simulink model "Opgave2_1"  (R2017a)
settings: Solver=VariableStepAuto  StartTime=0.0  StopTime=10.0  RelTol=1e-3
values from neighbouring files (symbols this model uses):
  b = 50    [Opgave2_1_script.m]
  F1 = 500    [Opgave2_1_script.m]
  m = 1000    [Opgave2_1_script.m]
settings Model: Creator=Sebastian  LastModifiedBy=Sebastian

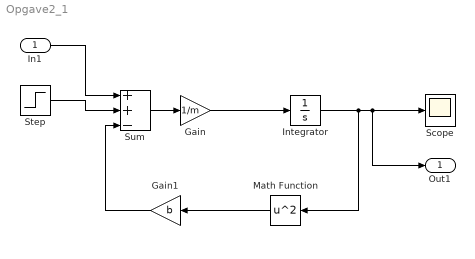
== system Opgave2_1 ==
  In1 : Inport
  Gain : Gain  Gain=1/m
  Gain1 : Gain  Gain=b
  Integrator : Integrator
  Math Function : Math  Operator=square  SaturateOnIntegerOverflow=on
  Scope : Scope
  Step : Step  After=F1  SampleTime=0
  Sum : Sum  Inputs=++-
  Out1 : Outport
  wires:
  Step/1 -> Sum/2
  Sum/1 -> Gain/1
  Gain/1 -> Integrator/1
  Integrator/1 -> Math Function/1, Out1/1, Scope/1
  Math Function/1 -> Gain1/1
  Gain1/1 -> Sum/3
  In1/1 -> Sum/1
